simulink model "GalacticSoupPhysical"  (R2025b)
settings: Solver=VariableStepAuto  StartTime=0.0  StopTime=10.0  RelTol=1e-3
settings Model: DataDictionary=GalacticSoupPhysicalInterfaces.sldd  Creator=sarah  LastModifiedBy=sarah

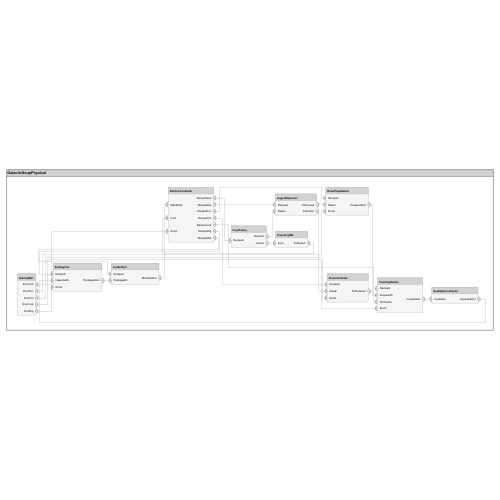
[thumbnail: Simulink's stored preview of the top-level diagram]
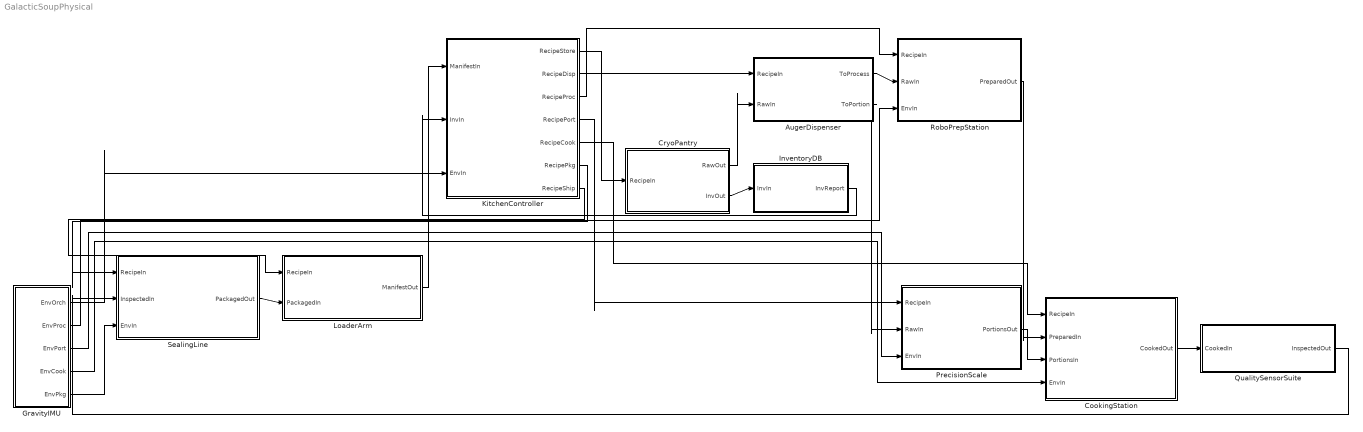
== system GalacticSoupPhysical ==
  AugerDispenser : Subsystem
      settings: PortSchema="{\"entries\":[{\"content\":{\"headerSize\":26,\"margin\":15,\"minimumSpacing\":25,\"sides\":[{\"content\":{\"connectorIds\":[\"In1\",\"In2\"]},\"type\":\"ConnectorPlacement.EquallySpacedRectSide\",\"uuid\":\"656a746b-557e-4d5f-bc1e-d3062d85d103\"},{\"content\":{\"connectorIds\":[\"Out1\",\"Out2\"],\"side\":\"RIGHT\"},\"type\":\"ConnectorPlacement.EquallySpacedRectSide\",\"uuid\":\"463d4e76-9095-47c1-86bc-6cb3ec56d7c4\"},{\"content\":{\"side\":\"TOP\"},\"type\":\"ConnectorPlacement.EquallySpacedRectSide\",\"uuid\":\"e2f1ba12-2af2-4ab2-99d2-a773f923d897\"}]},\"type\":\"ConnectorPlacement.EquallySpacedConnector\",\"uuid\":\"4f05f345-6ec4-40c2-8205-52053b27bd12\"}],\"packageUris\":[\"http://schema.mathworks.com/mf0/Connector/R2020b\"],\"version\":\"1.0\"}"
  CookingStation : Subsystem
      settings: PortSchema="{\"entries\":[{\"content\":{\"headerSize\":26,\"margin\":15,\"minimumSpacing\":25,\"sides\":[{\"content\":{\"connectorIds\":[\"In1\",\"In2\",\"In3\",\"In4\"]},\"type\":\"ConnectorPlacement.EquallySpacedRectSide\",\"uuid\":\"656a746b-557e-4d5f-bc1e-d3062d85d103\"},{\"content\":{\"connectorIds\":[\"Out1\"],\"side\":\"RIGHT\"},\"type\":\"ConnectorPlacement.EquallySpacedRectSide\",\"uuid\":\"463d4e76-9095-47c1-86bc-6cb3ec56d7c4\"},{\"content\":{\"side\":\"TOP\"},\"type\":\"ConnectorPlacement.EquallySpacedRectSide\",\"uuid\":\"e2f1ba12-2af2-4ab2-99d2-a773f923d897\"}]},\"type\":\"ConnectorPlacement.EquallySpacedConnector\",\"uuid\":\"4f05f345-6ec4-40c2-8205-52053b27bd12\"}],\"packageUris\":[\"http://schema.mathworks.com/mf0/Connector/R2020b\"],\"version\":\"1.0\"}"
  CryoPantry : Subsystem
      settings: PortSchema="{\"entries\":[{\"content\":{\"headerSize\":26,\"margin\":15,\"minimumSpacing\":25,\"sides\":[{\"content\":{\"connectorIds\":[\"In1\"]},\"type\":\"ConnectorPlacement.EquallySpacedRectSide\",\"uuid\":\"656a746b-557e-4d5f-bc1e-d3062d85d103\"},{\"content\":{\"connectorIds\":[\"Out1\",\"Out2\"],\"side\":\"RIGHT\"},\"type\":\"ConnectorPlacement.EquallySpacedRectSide\",\"uuid\":\"463d4e76-9095-47c1-86bc-6cb3ec56d7c4\"},{\"content\":{\"side\":\"TOP\"},\"type\":\"ConnectorPlacement.EquallySpacedRectSide\",\"uuid\":\"e2f1ba12-2af2-4ab2-99d2-a773f923d897\"}]},\"type\":\"ConnectorPlacement.EquallySpacedConnector\",\"uuid\":\"4f05f345-6ec4-40c2-8205-52053b27bd12\"}],\"packageUris\":[\"http://schema.mathworks.com/mf0/Connector/R2020b\"],\"version\":\"1.0\"}"
  GravityIMU : Subsystem
      settings: PortSchema="{\"entries\":[{\"content\":{\"headerSize\":26,\"margin\":15,\"minimumSpacing\":25,\"sides\":[{\"content\":{},\"type\":\"ConnectorPlacement.EquallySpacedRectSide\",\"uuid\":\"656a746b-557e-4d5f-bc1e-d3062d85d103\"},{\"content\":{\"connectorIds\":[\"Out1\",\"Out2\",\"Out3\",\"Out4\",\"Out5\"],\"side\":\"RIGHT\"},\"type\":\"ConnectorPlacement.EquallySpacedRectSide\",\"uuid\":\"463d4e76-9095-47c1-86bc-6cb3ec56d7c4\"},{\"content\":{\"side\":\"TOP\"},\"type\":\"ConnectorPlacement.EquallySpacedRectSide\",\"uuid\":\"e2f1ba12-2af2-4ab2-99d2-a773f923d897\"}]},\"type\":\"ConnectorPlacement.EquallySpacedConnector\",\"uuid\":\"4f05f345-6ec4-40c2-8205-52053b27bd12\"}],\"packageUris\":[\"http://schema.mathworks.com/mf0/Connector/R2020b\"],\"version\":\"1.0\"}"
  InventoryDB : Subsystem
      settings: PortSchema="{\"entries\":[{\"content\":{\"headerSize\":26,\"margin\":15,\"minimumSpacing\":25,\"sides\":[{\"content\":{\"connectorIds\":[\"In1\"]},\"type\":\"ConnectorPlacement.EquallySpacedRectSide\",\"uuid\":\"656a746b-557e-4d5f-bc1e-d3062d85d103\"},{\"content\":{\"connectorIds\":[\"Out1\"],\"side\":\"RIGHT\"},\"type\":\"ConnectorPlacement.EquallySpacedRectSide\",\"uuid\":\"463d4e76-9095-47c1-86bc-6cb3ec56d7c4\"},{\"content\":{\"side\":\"TOP\"},\"type\":\"ConnectorPlacement.EquallySpacedRectSide\",\"uuid\":\"e2f1ba12-2af2-4ab2-99d2-a773f923d897\"}]},\"type\":\"ConnectorPlacement.EquallySpacedConnector\",\"uuid\":\"4f05f345-6ec4-40c2-8205-52053b27bd12\"}],\"packageUris\":[\"http://schema.mathworks.com/mf0/Connector/R2020b\"],\"version\":\"1.0\"}"
  KitchenController : Subsystem
      settings: PortSchema="{\"entries\":[{\"content\":{\"headerSize\":26,\"margin\":15,\"minimumSpacing\":25,\"sides\":[{\"content\":{\"connectorIds\":[\"In1\",\"In2\",\"In3\"]},\"type\":\"ConnectorPlacement.EquallySpacedRectSide\",\"uuid\":\"656a746b-557e-4d5f-bc1e-d3062d85d103\"},{\"content\":{\"connectorIds\":[\"Out1\",\"Out2\",\"Out3\",\"Out4\",\"Out5\",\"Out6\",\"Out7\"],\"side\":\"RIGHT\"},\"type\":\"ConnectorPlacement.EquallySpacedRectSide\",\"uuid\":\"463d4e76-9095-47c1-86bc-6cb3ec56d7c4\"},{\"content\":{\"side\":\"TOP\"},\"type\":\"ConnectorPlacement.EquallySpacedRectSide\",\"uuid\":\"e2f1ba12-2af2-4ab2-99d2-a773f923d897\"}]},\"type\":\"ConnectorPlacement.EquallySpacedConnector\",\"uuid\":\"4f05f345-6ec4-40c2-8205-52053b27bd12\"}],\"packageUris\":[\"http://schema.mathworks.com/mf0/Connector/R2020b\"],\"version\":\"1.0\"}"
  LoaderArm : Subsystem
      settings: PortSchema="{\"entries\":[{\"content\":{\"headerSize\":26,\"margin\":15,\"minimumSpacing\":25,\"sides\":[{\"content\":{\"connectorIds\":[\"In1\",\"In2\"]},\"type\":\"ConnectorPlacement.EquallySpacedRectSide\",\"uuid\":\"656a746b-557e-4d5f-bc1e-d3062d85d103\"},{\"content\":{\"connectorIds\":[\"Out1\"],\"side\":\"RIGHT\"},\"type\":\"ConnectorPlacement.EquallySpacedRectSide\",\"uuid\":\"463d4e76-9095-47c1-86bc-6cb3ec56d7c4\"},{\"content\":{\"side\":\"TOP\"},\"type\":\"ConnectorPlacement.EquallySpacedRectSide\",\"uuid\":\"e2f1ba12-2af2-4ab2-99d2-a773f923d897\"}]},\"type\":\"ConnectorPlacement.EquallySpacedConnector\",\"uuid\":\"4f05f345-6ec4-40c2-8205-52053b27bd12\"}],\"packageUris\":[\"http://schema.mathworks.com/mf0/Connector/R2020b\"],\"version\":\"1.0\"}"
  PrecisionScale : Subsystem
      settings: PortSchema="{\"entries\":[{\"content\":{\"headerSize\":26,\"margin\":15,\"minimumSpacing\":25,\"sides\":[{\"content\":{\"connectorIds\":[\"In1\",\"In2\",\"In3\"]},\"type\":\"ConnectorPlacement.EquallySpacedRectSide\",\"uuid\":\"656a746b-557e-4d5f-bc1e-d3062d85d103\"},{\"content\":{\"connectorIds\":[\"Out1\"],\"side\":\"RIGHT\"},\"type\":\"ConnectorPlacement.EquallySpacedRectSide\",\"uuid\":\"463d4e76-9095-47c1-86bc-6cb3ec56d7c4\"},{\"content\":{\"side\":\"TOP\"},\"type\":\"ConnectorPlacement.EquallySpacedRectSide\",\"uuid\":\"e2f1ba12-2af2-4ab2-99d2-a773f923d897\"}]},\"type\":\"ConnectorPlacement.EquallySpacedConnector\",\"uuid\":\"4f05f345-6ec4-40c2-8205-52053b27bd12\"}],\"packageUris\":[\"http://schema.mathworks.com/mf0/Connector/R2020b\"],\"version\":\"1.0\"}"
  QualitySensorSuite : Subsystem
      settings: PortSchema="{\"entries\":[{\"content\":{\"headerSize\":26,\"margin\":15,\"minimumSpacing\":25,\"sides\":[{\"content\":{\"connectorIds\":[\"In1\"]},\"type\":\"ConnectorPlacement.EquallySpacedRectSide\",\"uuid\":\"656a746b-557e-4d5f-bc1e-d3062d85d103\"},{\"content\":{\"connectorIds\":[\"Out1\"],\"side\":\"RIGHT\"},\"type\":\"ConnectorPlacement.EquallySpacedRectSide\",\"uuid\":\"463d4e76-9095-47c1-86bc-6cb3ec56d7c4\"},{\"content\":{\"side\":\"TOP\"},\"type\":\"ConnectorPlacement.EquallySpacedRectSide\",\"uuid\":\"e2f1ba12-2af2-4ab2-99d2-a773f923d897\"}]},\"type\":\"ConnectorPlacement.EquallySpacedConnector\",\"uuid\":\"4f05f345-6ec4-40c2-8205-52053b27bd12\"}],\"packageUris\":[\"http://schema.mathworks.com/mf0/Connector/R2020b\"],\"version\":\"1.0\"}"
  RoboPrepStation : Subsystem
      settings: PortSchema="{\"entries\":[{\"content\":{\"headerSize\":26,\"margin\":15,\"minimumSpacing\":25,\"sides\":[{\"content\":{\"connectorIds\":[\"In1\",\"In2\",\"In3\"]},\"type\":\"ConnectorPlacement.EquallySpacedRectSide\",\"uuid\":\"656a746b-557e-4d5f-bc1e-d3062d85d103\"},{\"content\":{\"connectorIds\":[\"Out1\"],\"side\":\"RIGHT\"},\"type\":\"ConnectorPlacement.EquallySpacedRectSide\",\"uuid\":\"463d4e76-9095-47c1-86bc-6cb3ec56d7c4\"},{\"content\":{\"side\":\"TOP\"},\"type\":\"ConnectorPlacement.EquallySpacedRectSide\",\"uuid\":\"e2f1ba12-2af2-4ab2-99d2-a773f923d897\"}]},\"type\":\"ConnectorPlacement.EquallySpacedConnector\",\"uuid\":\"4f05f345-6ec4-40c2-8205-52053b27bd12\"}],\"packageUris\":[\"http://schema.mathworks.com/mf0/Connector/R2020b\"],\"version\":\"1.0\"}"
  SealingLine : Subsystem
      settings: PortSchema="{\"entries\":[{\"content\":{\"headerSize\":26,\"margin\":15,\"minimumSpacing\":25,\"sides\":[{\"content\":{\"connectorIds\":[\"In1\",\"In2\",\"In3\"]},\"type\":\"ConnectorPlacement.EquallySpacedRectSide\",\"uuid\":\"656a746b-557e-4d5f-bc1e-d3062d85d103\"},{\"content\":{\"connectorIds\":[\"Out1\"],\"side\":\"RIGHT\"},\"type\":\"ConnectorPlacement.EquallySpacedRectSide\",\"uuid\":\"463d4e76-9095-47c1-86bc-6cb3ec56d7c4\"},{\"content\":{\"side\":\"TOP\"},\"type\":\"ConnectorPlacement.EquallySpacedRectSide\",\"uuid\":\"e2f1ba12-2af2-4ab2-99d2-a773f923d897\"}]},\"type\":\"ConnectorPlacement.EquallySpacedConnector\",\"uuid\":\"4f05f345-6ec4-40c2-8205-52053b27bd12\"}],\"packageUris\":[\"http://schema.mathworks.com/mf0/Connector/R2020b\"],\"version\":\"1.0\"}"
  wires:
  LoaderArm/1(ManifestOut) -> KitchenController/1(ManifestIn)
  SealingLine/1(PackagedOut) -> LoaderArm/2(PackagedIn)
  GravityIMU/1(EnvOrch) -> KitchenController/3(EnvIn)
  GravityIMU/5(EnvPkg) -> SealingLine/3(EnvIn)
  GravityIMU/4(EnvCook) -> CookingStation/4(EnvIn)
  GravityIMU/3(EnvPort) -> PrecisionScale/3(EnvIn)
  GravityIMU/2(EnvProc) -> RoboPrepStation/3(EnvIn)
  KitchenController/1(RecipeStore) -> CryoPantry/1(RecipeIn)
  KitchenController/2(RecipeDisp) -> AugerDispenser/1(RecipeIn)
  KitchenController/3(RecipeProc) -> RoboPrepStation/1(RecipeIn)
  KitchenController/4(RecipePort) -> PrecisionScale/1(RecipeIn)
  KitchenController/5(RecipeCook) -> CookingStation/1(RecipeIn)
  KitchenController/6(RecipePkg) -> SealingLine/1(RecipeIn)
  KitchenController/7(RecipeShip) -> LoaderArm/1(RecipeIn)
  CryoPantry/1(RawOut) -> AugerDispenser/2(RawIn)
  CryoPantry/2(InvOut) -> InventoryDB/1(InvIn)
  AugerDispenser/1(ToProcess) -> RoboPrepStation/2(RawIn)
  AugerDispenser/2(ToPortion) -> PrecisionScale/2(RawIn)
  InventoryDB/1(InvReport) -> KitchenController/2(InvIn)
  RoboPrepStation/1(PreparedOut) -> CookingStation/2(PreparedIn)
  PrecisionScale/1(PortionsOut) -> CookingStation/3(PortionsIn)
  CookingStation/1(CookedOut) -> QualitySensorSuite/1(CookedIn)
  QualitySensorSuite/1(InspectedOut) -> SealingLine/2(InspectedIn)

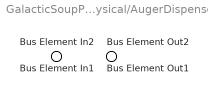
== system GalacticSoupPhysical/AugerDispenser ==
  Bus Element In1 : Inport  PortName=RecipeIn
  Bus Element In2 : Inport  Port=2  PortName=RawIn
  Bus Element Out1 : Outport  PortName=ToProcess
  Bus Element Out2 : Outport  Port=2  PortName=ToPortion

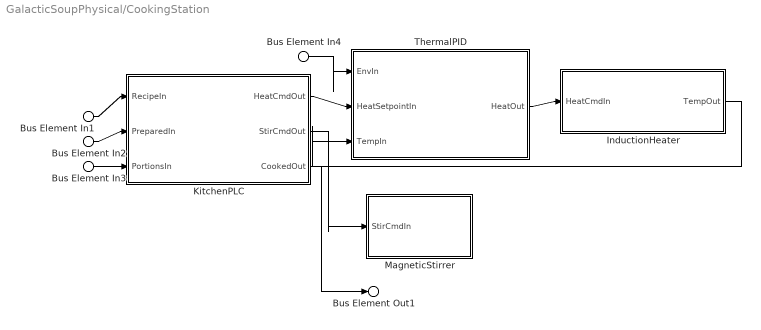
== system GalacticSoupPhysical/CookingStation ==
  Bus Element In1 : Inport  PortName=RecipeIn
  Bus Element In2 : Inport  Port=2  PortName=PreparedIn
  Bus Element In3 : Inport  Port=3  PortName=PortionsIn
  Bus Element In4 : Inport  Port=4  PortName=EnvIn
  InductionHeater : Subsystem
      settings: PortSchema="{\"entries\":[{\"content\":{\"headerSize\":26,\"margin\":15,\"minimumSpacing\":25,\"sides\":[{\"content\":{\"connectorIds\":[\"In1\"]},\"type\":\"ConnectorPlacement.EquallySpacedRectSide\",\"uuid\":\"656a746b-557e-4d5f-bc1e-d3062d85d103\"},{\"content\":{\"connectorIds\":[\"Out1\"],\"side\":\"RIGHT\"},\"type\":\"ConnectorPlacement.EquallySpacedRectSide\",\"uuid\":\"463d4e76-9095-47c1-86bc-6cb3ec56d7c4\"},{\"content\":{\"side\":\"TOP\"},\"type\":\"ConnectorPlacement.EquallySpacedRectSide\",\"uuid\":\"e2f1ba12-2af2-4ab2-99d2-a773f923d897\"}]},\"type\":\"ConnectorPlacement.EquallySpacedConnector\",\"uuid\":\"4f05f345-6ec4-40c2-8205-52053b27bd12\"}],\"packageUris\":[\"http://schema.mathworks.com/mf0/Connector/R2020b\"],\"version\":\"1.0\"}"
  KitchenPLC : Subsystem
      settings: PortSchema="{\"entries\":[{\"content\":{\"headerSize\":26,\"margin\":15,\"minimumSpacing\":25,\"sides\":[{\"content\":{\"connectorIds\":[\"In1\",\"In2\",\"In3\"]},\"type\":\"ConnectorPlacement.EquallySpacedRectSide\",\"uuid\":\"656a746b-557e-4d5f-bc1e-d3062d85d103\"},{\"content\":{\"connectorIds\":[\"Out1\",\"Out2\",\"Out3\"],\"side\":\"RIGHT\"},\"type\":\"ConnectorPlacement.EquallySpacedRectSide\",\"uuid\":\"463d4e76-9095-47c1-86bc-6cb3ec56d7c4\"},{\"content\":{\"side\":\"TOP\"},\"type\":\"ConnectorPlacement.EquallySpacedRectSide\",\"uuid\":\"e2f1ba12-2af2-4ab2-99d2-a773f923d897\"}]},\"type\":\"ConnectorPlacement.EquallySpacedConnector\",\"uuid\":\"4f05f345-6ec4-40c2-8205-52053b27bd12\"}],\"packageUris\":[\"http://schema.mathworks.com/mf0/Connector/R2020b\"],\"version\":\"1.0\"}"
  MagneticStirrer : Subsystem
      settings: PortSchema="{\"entries\":[{\"content\":{\"headerSize\":26,\"margin\":15,\"minimumSpacing\":25,\"sides\":[{\"content\":{\"connectorIds\":[\"In1\"]},\"type\":\"ConnectorPlacement.EquallySpacedRectSide\",\"uuid\":\"656a746b-557e-4d5f-bc1e-d3062d85d103\"},{\"content\":{\"side\":\"RIGHT\"},\"type\":\"ConnectorPlacement.EquallySpacedRectSide\",\"uuid\":\"463d4e76-9095-47c1-86bc-6cb3ec56d7c4\"},{\"content\":{\"side\":\"TOP\"},\"type\":\"ConnectorPlacement.EquallySpacedRectSide\",\"uuid\":\"e2f1ba12-2af2-4ab2-99d2-a773f923d897\"}]},\"type\":\"ConnectorPlacement.EquallySpacedConnector\",\"uuid\":\"4f05f345-6ec4-40c2-8205-52053b27bd12\"}],\"packageUris\":[\"http://schema.mathworks.com/mf0/Connector/R2020b\"],\"version\":\"1.0\"}"
  ThermalPID : Subsystem
      settings: PortSchema="{\"entries\":[{\"content\":{\"headerSize\":26,\"margin\":15,\"minimumSpacing\":25,\"sides\":[{\"content\":{\"connectorIds\":[\"In1\",\"In2\",\"In3\"]},\"type\":\"ConnectorPlacement.EquallySpacedRectSide\",\"uuid\":\"656a746b-557e-4d5f-bc1e-d3062d85d103\"},{\"content\":{\"connectorIds\":[\"Out1\"],\"side\":\"RIGHT\"},\"type\":\"ConnectorPlacement.EquallySpacedRectSide\",\"uuid\":\"463d4e76-9095-47c1-86bc-6cb3ec56d7c4\"},{\"content\":{\"side\":\"TOP\"},\"type\":\"ConnectorPlacement.EquallySpacedRectSide\",\"uuid\":\"e2f1ba12-2af2-4ab2-99d2-a773f923d897\"}]},\"type\":\"ConnectorPlacement.EquallySpacedConnector\",\"uuid\":\"4f05f345-6ec4-40c2-8205-52053b27bd12\"}],\"packageUris\":[\"http://schema.mathworks.com/mf0/Connector/R2020b\"],\"version\":\"1.0\"}"
  Bus Element Out1 : Outport  PortName=CookedOut
  wires:
  Bus Element In1/1 -> KitchenPLC/1(RecipeIn)
  Bus Element In3/1 -> KitchenPLC/3(PortionsIn)
  Bus Element In2/1 -> KitchenPLC/2(PreparedIn)
  Bus Element In4/1 -> ThermalPID/1(EnvIn)
  KitchenPLC/2(StirCmdOut) -> MagneticStirrer/1(StirCmdIn)
  KitchenPLC/1(HeatCmdOut) -> ThermalPID/2(HeatSetpointIn)
  ThermalPID/1(HeatOut) -> InductionHeater/1(HeatCmdIn)
  KitchenPLC/3(CookedOut) -> Bus Element Out1/1
  InductionHeater/1(TempOut) -> ThermalPID/3(TempIn)

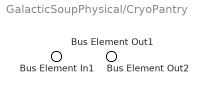
== system GalacticSoupPhysical/CryoPantry ==
  Bus Element In1 : Inport  PortName=RecipeIn
  Bus Element Out1 : Outport  PortName=RawOut
  Bus Element Out2 : Outport  Port=2  PortName=InvOut

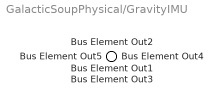
== system GalacticSoupPhysical/GravityIMU ==
  Bus Element Out1 : Outport  PortName=EnvOrch
  Bus Element Out2 : Outport  Port=2  PortName=EnvProc
  Bus Element Out3 : Outport  Port=3  PortName=EnvPort
  Bus Element Out4 : Outport  Port=4  PortName=EnvCook
  Bus Element Out5 : Outport  Port=5  PortName=EnvPkg

== system GalacticSoupPhysical/InventoryDB ==
  Bus Element In1 : Inport  PortName=InvIn
  Bus Element Out1 : Outport  PortName=InvReport

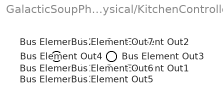
== system GalacticSoupPhysical/KitchenController ==
  Bus Element In1 : Inport  PortName=ManifestIn
  Bus Element In2 : Inport  Port=2  PortName=InvIn
  Bus Element In3 : Inport  Port=3  PortName=EnvIn
  Bus Element Out1 : Outport  PortName=RecipeStore
  Bus Element Out2 : Outport  Port=2  PortName=RecipeDisp
  Bus Element Out3 : Outport  Port=3  PortName=RecipeProc
  Bus Element Out4 : Outport  Port=4  PortName=RecipePort
  Bus Element Out5 : Outport  Port=5  PortName=RecipeCook
  Bus Element Out6 : Outport  Port=6  PortName=RecipePkg
  Bus Element Out7 : Outport  Port=7  PortName=RecipeShip

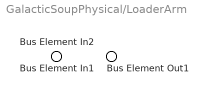
== system GalacticSoupPhysical/LoaderArm ==
  Bus Element In1 : Inport  PortName=RecipeIn
  Bus Element In2 : Inport  Port=2  PortName=PackagedIn
  Bus Element Out1 : Outport  PortName=ManifestOut

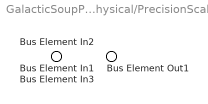
== system GalacticSoupPhysical/PrecisionScale ==
  Bus Element In1 : Inport  PortName=RecipeIn
  Bus Element In2 : Inport  Port=2  PortName=RawIn
  Bus Element In3 : Inport  Port=3  PortName=EnvIn
  Bus Element Out1 : Outport  PortName=PortionsOut

== system GalacticSoupPhysical/QualitySensorSuite ==
  Bus Element In1 : Inport  PortName=CookedIn
  Bus Element Out1 : Outport  PortName=InspectedOut

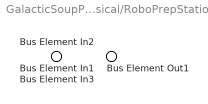
== system GalacticSoupPhysical/RoboPrepStation ==
  Bus Element In1 : Inport  PortName=RecipeIn
  Bus Element In2 : Inport  Port=2  PortName=RawIn
  Bus Element In3 : Inport  Port=3  PortName=EnvIn
  Bus Element Out1 : Outport  PortName=PreparedOut

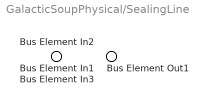
== system GalacticSoupPhysical/SealingLine ==
  Bus Element In1 : Inport  PortName=RecipeIn
  Bus Element In2 : Inport  Port=2  PortName=InspectedIn
  Bus Element In3 : Inport  Port=3  PortName=EnvIn
  Bus Element Out1 : Outport  PortName=PackagedOut

== system GalacticSoupPhysical/CookingStation/InductionHeater ==
  Bus Element In1 : Inport  PortName=HeatCmdIn
  Bus Element Out1 : Outport  PortName=TempOut

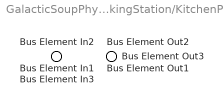
== system GalacticSoupPhysical/CookingStation/KitchenPLC ==
  Bus Element In1 : Inport  PortName=RecipeIn
  Bus Element In2 : Inport  Port=2  PortName=PreparedIn
  Bus Element In3 : Inport  Port=3  PortName=PortionsIn
  Bus Element Out1 : Outport  PortName=HeatCmdOut
  Bus Element Out2 : Outport  Port=2  PortName=StirCmdOut
  Bus Element Out3 : Outport  Port=3  PortName=CookedOut

== system GalacticSoupPhysical/CookingStation/MagneticStirrer ==
  Bus Element In1 : Inport  PortName=StirCmdIn

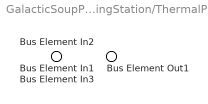
== system GalacticSoupPhysical/CookingStation/ThermalPID ==
  Bus Element In1 : Inport  PortName=EnvIn
  Bus Element In2 : Inport  Port=2  PortName=HeatSetpointIn
  Bus Element In3 : Inport  Port=3  PortName=TempIn
  Bus Element Out1 : Outport  PortName=HeatOut
